simulink model "gm_sampleModel1811_5_sub"  (R2023a)
settings: Solver=VariableStepAuto  StartTime=0.0  StopTime=10.0  RelTol=1e-3
libraries: simulink x5
settings Model: Creator=user1  LastModifiedBy=user1
settings OptimizationCC: BlockReduction=off  ConditionallyExecuteInputs=off
settings DebuggingCC: InheritedTsInSrcMsg=none

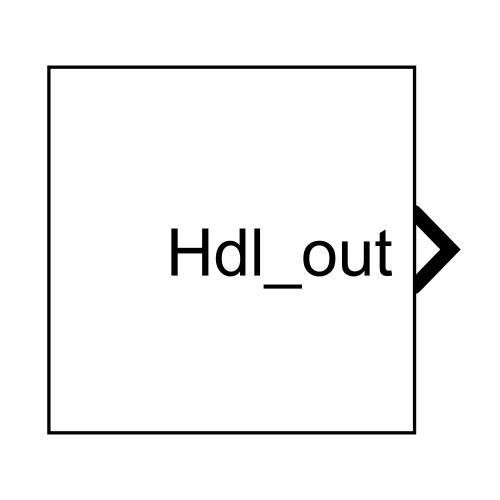
[thumbnail: Simulink's stored preview of the top-level diagram]
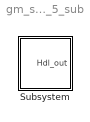
== system gm_sampleModel1811_5_sub ==
  Subsystem : Subsystem

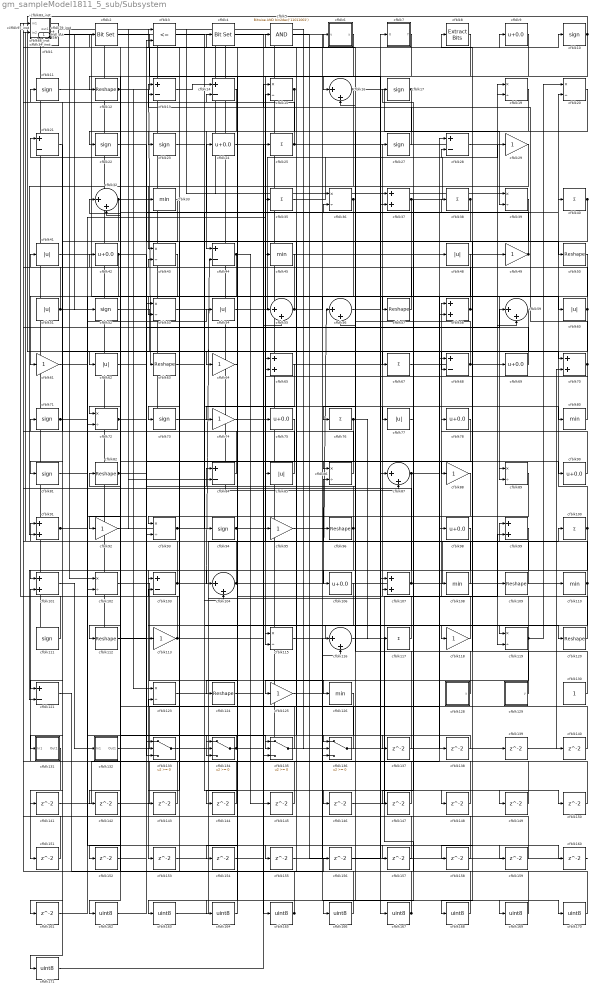
== system gm_sampleModel1811_5_sub/Subsystem ==
  cfblk1 : simulink/Logic and Bit Operations/Detect Decrease  vinit=0.0  OutDataTypeStr=uint8
      settings: LibrarySourceBlock=|
      | hdlsllib/Logic and Bit
      | Operations/Detect
      | Decrease
  cfblk{10..11,17,22..23,27,52,71,73,81,94,111} (12 alike) : Signum
  cfblk{25,35,38,40,67,76,100,117} (8 alike) : Sum  Inputs=+  OutDataTypeStr=uint8
  cfblk{37,58,65,70,91,99,101,107} (8 alike) : Sum  OutDataTypeStr=uint8
  cfblk{15,19..20,36,39,43,53,72,86,89,93,102,115,119,123} (15 alike) : Product  Inputs=*/  OutDataTypeStr=uint8  RndMeth=Zero  SaturateOnIntegerOverflow=on
  cfblk{13..14,21,28,44,68,84,103,121} (9 alike) : Sum  Inputs=+-  OutDataTypeStr=uint8
  cfblk{16,32,55..56,59,87,104,116} (8 alike) : Sum  Inputs=|++  OutDataTypeStr=uint8
  cfblk105_inst : Subsystem
  cfblk{9,24,42,69,75,78,90,98,106} (9 alike) : Bias  Bias=0.0  SaturateOnIntegerOverflow=off
  cfblk{33,45,80,108,110,126} (6 alike) : MinMax  OutDataTypeStr=uint8
  cfblk{12,50,57,63,82,96,109,112,120,124} (10 alike) : Reshape
  cfblk{29,49,61,64,74,88,92,95,113,118,125} (11 alike) : Gain  OutDataTypeStr=uint8
  cfblk114_inst : Subsystem
  cfblk122_inst : Subsystem
  cfblk128 : Subsystem  mask(Counter Free-Running){NumBits=double(16), tsamp=double(-1)}
      mask prompts: NumBits "Simulink:masks:NumberOfBits_MP"; tsamp "Simulink:masks:SampleTime_MP"
      mask help: Simulink:masks:CounterFreeRunning_MD
  cfblk129 : Subsystem  mask(Counter Limited){uplimit=double(7), tsamp=double(-1)}
      mask prompts: uplimit "Simulink:masks:UpperLimit_MP"; tsamp "Simulink:masks:SampleTime_MP"
      mask help: Simulink:masks:CounterLimited_MD
      mask init:
      | nbits = double(8);
      | tsamp = double(-1);
      | uplimit = double(7);
  cfblk130 : Constant  OutDataTypeStr=uint8  SampleTime=-1
  cfblk131 : Subsystem
  cfblk132 : Subsystem
  cfblk{133..136} (4 alike) : Switch  OutDataTypeStr=uint8  SaturateOnIntegerOverflow=off  InputSameDT=off
  cfblk{137..161} (25 alike) : Delay  SampleTime=1
  cfblk{162..171} (10 alike) : DataTypeConversion  OutDataTypeStr=uint8  SaturateOnIntegerOverflow=off  RndMeth=Floor
  cfblk18_inst : Subsystem
  cfblk2 : simulink/Logic and Bit Operations/Bit Set  iBit=0
      settings: LibrarySourceBlock=|
      | hdlsllib/Logic and Bit
      | Operations/Bit Set
  cfblk26_inst : Subsystem
  cfblk3 : RelationalOperator  Operator=<=  OutDataTypeStr=boolean  InputSameDT=off
  cfblk30_inst : Subsystem
  cfblk31_inst : Subsystem
  cfblk34_inst : Subsystem
  cfblk4 : simulink/Logic and Bit Operations/Bit Set  iBit=0
      settings: LibrarySourceBlock=|
      | hdlsllib/Logic and Bit
      | Operations/Bit Set
  cfblk{41,48,51,54,60,62,77,85} (8 alike) : Abs  OutDataTypeStr=uint8  SaturateOnIntegerOverflow=off
  cfblk5 : simulink/Logic and Bit Operations/Bitwise Operator  logicop=AND  UseBitMask=on  BitMask=bin2dec('11011001')  BitMaskRealWorld=Stored Integer
      settings: LibrarySourceBlock=|
      | hdlsllib/Logic and Bit
      | Operations/Bitwise
      | Operator
  cfblk6 : Subsystem  mask(Compare To Zero){relop=<=, OutDataTypeStr=uint8, ZeroCross=on}
      mask prompts: relop "Simulink:masks:Operator_MP"; OutDataTypeStr "Simulink:masks:OutputDataType_MP"; ZeroCross "Simulink:masks:EnableZerocrossingDetection_MP"
      mask help: Simulink:masks:CompareToZero_MD
      mask init:
      | OutDataTypeStr = 'uint8';
      | ZeroCross = 'on';
      | blkName = 'sampleModel1811_5_sub/Subsystem/cfblk6';
      | relop = '<=';
      | setValue = 'fixdt(0, 8)';
      mask TypeOptions relop: == | ~= | < | <= | >= | >
      mask TypeOptions OutDataTypeStr: Simulink:masks:uint8 | Simulink:masks:boolean
      mask Callback ZeroCross: sl('zeroCrossEnable', gcbh);
      mask Display: disp([relop,' 0'])
  cfblk66_inst : Subsystem
  cfblk7 : Subsystem  mask(Detect Fall Nonpositive){vinit=double(0), InputProcessing=Elements as channels (sample based), OutDataTypeStr=uint8}
      mask prompts: vinit "Simulink:masks:InitialCondition_MP"; InputProcessing "Simulink:masks:InputProcessing_MP"; OutDataTypeStr "Simulink:masks:OutputDataType_MP"
      mask help: Simulink:masks:DetectFallNonpositive_MD
      mask init:
      | InputProcessing = 'Elements as channels (sample based)';
      | OutDataTypeStr = 'uint8';
      | vinit = double(0);
      mask TypeOptions InputProcessing: Simulink:masks:ColumnsAsChannelsFrameBased | Simulink:masks:ElementsAsChannelsSampleBased
      mask TypeOptions OutDataTypeStr: Simulink:masks:uint8 | Simulink:masks:boolean
      mask Display: fprintf('U <= 0\n&  NOT\nU/z <= 0')
  cfblk79_inst : Subsystem
  cfblk8 : simulink/Logic and Bit Operations/Extract Bits  bitsToExtract=Upper half  numBits=8  bitIdxRange=[0 7]  outScalingMode=Preserve fixed-point scaling
      settings: LibrarySourceBlock=|
      | hdlsllib/Logic and Bit
      | Operations/Extract Bits
  cfblk83_inst : Subsystem
  cfblk97_inst : Subsystem
  Hdl_out : Outport  OutDataTypeStr=uint8  SampleTime=1
  wires:
  cfblk1/1 -> cfblk52/1, cfblk89/2
  cfblk10/1 -> cfblk62/1, cfblk115/2
  cfblk100/1 -> cfblk20/2, cfblk153/1
  cfblk101/1 -> cfblk132/1(In1)
  cfblk102/1 -> cfblk126/1
  cfblk103/1 -> cfblk44/2, cfblk31_inst/2(in2)
  cfblk104/1 -> cfblk56/1, cfblk18_inst/2(in2)
  cfblk105_inst/1(out1) -> cfblk122_inst/2(in2)
  cfblk106/1 -> cfblk113/1
  cfblk107/1 -> cfblk26_inst/2(in2), cfblk100/1
  cfblk108/1 -> cfblk15/2
  cfblk109/1 -> cfblk91/1
  cfblk11/1 -> cfblk109/1
  cfblk110/1 -> cfblk56/2, cfblk86/2, cfblk125/1
  cfblk111/1 -> cfblk83_inst/1(in1)
  cfblk112/1 -> cfblk10/1
  cfblk113/1 -> cfblk105_inst/2(in2), cfblk157/1, Hdl_out/1
  cfblk114_inst/1(out1) -> cfblk75/1, cfblk66_inst/2(in2), cfblk49/1
  cfblk115/1 -> cfblk118/1
  cfblk116/1 -> cfblk163/1
  cfblk117/1 -> cfblk27/1
  cfblk118/1 -> cfblk58/1
  cfblk119/1 -> cfblk135/2, cfblk107/2, cfblk20/1
  cfblk12/1 -> cfblk63/1, cfblk123/1, cfblk6/1(u)
  cfblk120/1 -> cfblk71/1
  cfblk121/1 -> cfblk156/1
  cfblk122_inst/1(out1) -> cfblk94/1, cfblk37/1
  cfblk123/1 -> cfblk99/1
  cfblk124/1 -> cfblk25/1
  cfblk125/1 -> cfblk116/2
  cfblk126/1 -> cfblk152/1
  cfblk128/1(y) -> cfblk84/1
  cfblk129/1(y) -> cfblk78/1
  cfblk13/1 -> cfblk14/1
  cfblk130/1 -> cfblk16/2
  cfblk131/1(Out1) -> cfblk151/1
  cfblk132/1(Out1) -> cfblk108/1
  cfblk133/1 -> cfblk85/1
  cfblk134/1 -> cfblk133/2, cfblk160/1
  cfblk135/1 -> cfblk43/2
  cfblk136/1 -> cfblk32/1
  cfblk137/1 -> cfblk97_inst/2(in2)
  cfblk138/1 -> cfblk136/1
  cfblk139/1 -> cfblk70/2
  cfblk14/1 -> cfblk72/1
  cfblk140/1 -> cfblk123/2
  cfblk141/1 -> cfblk28/1
  cfblk142/1 -> cfblk116/1
  cfblk143/1 -> cfblk83_inst/2(in2)
  cfblk144/1 -> cfblk32/2
  cfblk145/1 -> cfblk30_inst/2(in2)
  cfblk146/1 -> cfblk99/2
  cfblk147/1 -> cfblk101/2
  cfblk148/1 -> cfblk34_inst/2(in2)
  cfblk149/1 -> cfblk122_inst/1(in1)
  cfblk15/1 -> cfblk22/1, cfblk64/1
  cfblk150/1 -> cfblk14/2
  cfblk151/1 -> cfblk26_inst/1(in1)
  cfblk152/1 -> cfblk59/1
  cfblk153/1 -> cfblk107/1
  cfblk154/1 -> cfblk55/2
  cfblk155/1 -> cfblk136/3
  cfblk156/1 -> cfblk87/1
  cfblk157/1 -> cfblk3/1
  cfblk158/1 -> cfblk13/1
  cfblk159/1 -> cfblk79_inst/2(in2)
  cfblk16/1 -> cfblk43/1, cfblk39/2
  cfblk160/1 -> cfblk1/1
  cfblk161/1 -> cfblk72/2
  cfblk162/1 -> cfblk9/1
  cfblk163/1 -> cfblk7/1(U)
  cfblk164/1 -> cfblk4/1
  cfblk165/1 -> cfblk34_inst/1(in1), cfblk114_inst/1(in1)
  cfblk166/1 -> cfblk2/1
  cfblk167/1 -> cfblk82/1, cfblk133/1, cfblk103/2
  cfblk168/1 -> cfblk5/1
  cfblk169/1 -> cfblk17/1
  cfblk17/1 -> cfblk37/2, cfblk76/1
  cfblk170/1 -> cfblk97_inst/1(in1)
  cfblk171/1 -> cfblk95/1
  cfblk18_inst/1(out1) -> cfblk39/1
  cfblk19/1 -> cfblk44/1
  cfblk2/1 -> cfblk167/1
  cfblk20/1 -> cfblk23/1
  cfblk21/1 -> cfblk81/1
  cfblk22/1 -> cfblk50/1
  cfblk23/1 -> cfblk104/2
  cfblk24/1 -> cfblk89/1
  cfblk25/1 -> cfblk90/1, cfblk79_inst/1(in1)
  cfblk26_inst/1(out1) -> cfblk84/2
  cfblk27/1 -> cfblk15/1
  cfblk28/1 -> cfblk119/2
  cfblk29/1 -> cfblk91/2
  cfblk3/1 -> cfblk65/1
  cfblk30_inst/1(out1) -> cfblk111/1, cfblk102/1
  cfblk31_inst/1(out1) -> cfblk105_inst/1(in1), cfblk29/1
  cfblk32/1 -> cfblk161/1, cfblk33/1
  cfblk33/1 -> cfblk171/1
  cfblk34_inst/1(out1) -> cfblk69/1
  cfblk35/1 -> cfblk28/2
  cfblk36/1 -> cfblk102/2, cfblk131/1(In1)
  cfblk37/1 -> cfblk57/1, cfblk19/2, cfblk147/1
  cfblk38/1 -> cfblk103/1, cfblk115/1
  cfblk39/1 -> cfblk68/2
  cfblk4/1 -> cfblk165/1
  cfblk40/1 -> cfblk96/1, cfblk106/1
  cfblk41/1 -> cfblk98/1
  cfblk42/1 -> cfblk60/1, cfblk59/2, cfblk134/3, cfblk121/1, cfblk61/1
  cfblk43/1 -> cfblk141/1
  cfblk44/1 -> cfblk73/1, cfblk145/1, cfblk144/1
  cfblk45/1 -> cfblk74/1
  cfblk48/1 -> cfblk136/2
  cfblk49/1 -> cfblk24/1, cfblk21/1
  cfblk5/1 -> cfblk169/1
  cfblk50/1 -> cfblk93/1
  cfblk51/1 -> cfblk114_inst/2(in2), cfblk67/1
  cfblk52/1 -> cfblk70/1
  cfblk53/1 -> cfblk138/1
  cfblk54/1 -> cfblk19/1
  cfblk55/1 -> cfblk58/2, cfblk53/2
  cfblk56/1 -> cfblk80/1
  cfblk57/1 -> cfblk45/1
  cfblk58/1 -> cfblk42/1, cfblk168/1
  cfblk59/1 -> cfblk101/1
  cfblk6/1(y) -> cfblk104/1
  cfblk60/1 -> cfblk18_inst/1(in1), cfblk158/1
  cfblk61/1 -> cfblk159/1
  cfblk62/1 -> cfblk86/1
  cfblk63/1 -> cfblk77/1
  cfblk64/1 -> cfblk164/1
  cfblk65/1 -> cfblk124/1
  cfblk66_inst/1(out1) -> cfblk31_inst/1(in1), cfblk36/1
  cfblk67/1 -> cfblk120/1
  cfblk68/1 -> cfblk41/1, cfblk88/1
  cfblk69/1 -> cfblk30_inst/1(in1)
  cfblk7/1(Y) -> cfblk162/1
  cfblk70/1 -> cfblk65/2, cfblk13/2
  cfblk71/1 -> cfblk93/2, cfblk35/1
  cfblk72/1 -> cfblk3/2, cfblk38/1
  cfblk73/1 -> cfblk146/1
  cfblk74/1 -> cfblk148/1
  cfblk75/1 -> cfblk92/1
  cfblk76/1 -> cfblk134/1, cfblk117/1
  cfblk77/1 -> cfblk137/1
  cfblk78/1 -> cfblk135/3
  cfblk79_inst/1(out1) -> cfblk87/2
  cfblk8/1 -> cfblk16/1
  cfblk80/1 -> cfblk68/1
  cfblk81/1 -> cfblk155/1
  cfblk82/1 -> cfblk133/3, cfblk112/1
  cfblk83_inst/1(out1) -> cfblk51/1, cfblk21/2, cfblk140/1, cfblk139/1
  cfblk84/1 -> cfblk66_inst/1(in1)
  cfblk85/1 -> cfblk11/1
  cfblk86/1 -> cfblk55/1
  cfblk87/1 -> cfblk48/1, cfblk134/2
  cfblk88/1 -> cfblk143/1
  cfblk89/1 -> cfblk154/1
  cfblk9/1 -> cfblk12/1
  cfblk90/1 -> cfblk8/1
  cfblk91/1 -> cfblk54/1, cfblk135/1
  cfblk92/1 -> cfblk40/1
  cfblk93/1 -> cfblk36/2, cfblk119/1
  cfblk94/1 -> cfblk150/1, cfblk149/1
  cfblk95/1 -> cfblk170/1
  cfblk96/1 -> cfblk121/2, cfblk53/1
  cfblk97_inst/1(out1) -> cfblk110/1
  cfblk98/1 -> cfblk142/1
  cfblk99/1 -> cfblk166/1

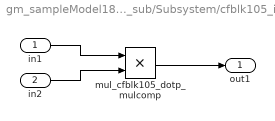
== system gm_sampleModel1811_5_sub/Subsystem/cfblk105_inst ==
  in1 : Inport  OutDataTypeStr=uint8  SampleTime=1
  in2 : Inport  Port=2  OutDataTypeStr=uint8  SampleTime=1
  mul_cfblk105_dotp_mulcomp : Product  Inputs=**  OutDataTypeStr=uint8  SampleTime=1
  out1 : Outport  OutDataTypeStr=uint8  SampleTime=1
  wires:
  in1/1 -> mul_cfblk105_dotp_mulcomp/1
  in2/1 -> mul_cfblk105_dotp_mulcomp/2
  mul_cfblk105_dotp_mulcomp/1 -> out1/1

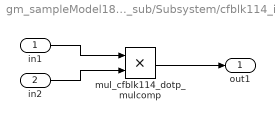
== system gm_sampleModel1811_5_sub/Subsystem/cfblk114_inst ==
  in1 : Inport  OutDataTypeStr=uint8  SampleTime=1
  in2 : Inport  Port=2  OutDataTypeStr=uint8  SampleTime=1
  mul_cfblk114_dotp_mulcomp : Product  Inputs=**  OutDataTypeStr=uint8  SampleTime=1
  out1 : Outport  OutDataTypeStr=uint8  SampleTime=1
  wires:
  in1/1 -> mul_cfblk114_dotp_mulcomp/1
  in2/1 -> mul_cfblk114_dotp_mulcomp/2
  mul_cfblk114_dotp_mulcomp/1 -> out1/1

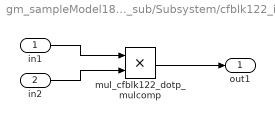
== system gm_sampleModel1811_5_sub/Subsystem/cfblk122_inst ==
  in1 : Inport  OutDataTypeStr=uint8  SampleTime=1
  in2 : Inport  Port=2  OutDataTypeStr=uint8  SampleTime=1
  mul_cfblk122_dotp_mulcomp : Product  Inputs=**  OutDataTypeStr=uint8  SampleTime=1
  out1 : Outport  OutDataTypeStr=uint8  SampleTime=1
  wires:
  in1/1 -> mul_cfblk122_dotp_mulcomp/1
  in2/1 -> mul_cfblk122_dotp_mulcomp/2
  mul_cfblk122_dotp_mulcomp/1 -> out1/1

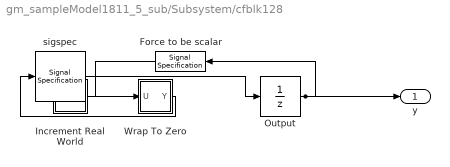
== system gm_sampleModel1811_5_sub/Subsystem/cfblk128 ==
  Force to be scalar : SignalSpecification  DisableCoverage=on  Dimensions=1
  Increment Real World : Subsystem  mask(Real World Value Increment){}
      mask help: Simulink:masks:RealWorldValueIncrement_MD
      mask Display: disp('V++')
  Output : UnitDelay  InitialCondition=0.0  SampleTime=tsamp  HasFrameUpgradeWarning=on
  Wrap To Zero : Subsystem  mask(Wrap To Zero){Threshold=double(65535)}
      mask prompts: Threshold "Simulink:masks:Threshold_MP"
      mask help: Simulink:masks:WrapToZero_MD
  sigspec : SignalSpecification  OutDataTypeStr=uint16  Dimensions=1
  y : Outport  SampleTime=1
  wires:
  Force to be scalar/1 -> Increment Real World/1(u)
  Increment Real World/1(y) -> Wrap To Zero/1(U)
  Output/1 -> Force to be scalar/1, y/1
  Wrap To Zero/1(Y) -> sigspec/1
  sigspec/1 -> Output/1

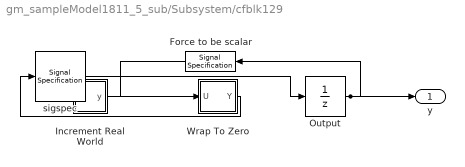
== system gm_sampleModel1811_5_sub/Subsystem/cfblk129 ==
  Force to be scalar : SignalSpecification  DisableCoverage=on  Dimensions=1
  Increment Real World : Subsystem  mask(Real World Value Increment){}
      mask help: Simulink:masks:RealWorldValueIncrement_MD
      mask Display: disp('V++')
  Output : UnitDelay  InitialCondition=0.0  SampleTime=tsamp  HasFrameUpgradeWarning=on
  Wrap To Zero : Subsystem  mask(Wrap To Zero){Threshold=double(7)}
      mask prompts: Threshold "Simulink:masks:Threshold_MP"
      mask help: Simulink:masks:WrapToZero_MD
  sigspec : SignalSpecification  OutDataTypeStr=uint8  Dimensions=1
  y : Outport  SampleTime=1
  wires:
  Force to be scalar/1 -> Increment Real World/1(u)
  Increment Real World/1(y) -> Wrap To Zero/1(U)
  Output/1 -> Force to be scalar/1, y/1
  Wrap To Zero/1(Y) -> sigspec/1
  sigspec/1 -> Output/1

== system gm_sampleModel1811_5_sub/Subsystem/cfblk131 ==
  In1 : Inport  OutDataTypeStr=uint8  PortDimensions=1  SampleTime=1
  Out1 : Outport  SampleTime=1
  wires:
  In1/1 -> Out1/1

== system gm_sampleModel1811_5_sub/Subsystem/cfblk132 ==
  In1 : Inport  OutDataTypeStr=uint8  PortDimensions=1  SampleTime=1
  Out1 : Outport  SampleTime=1
  wires:
  In1/1 -> Out1/1

== system gm_sampleModel1811_5_sub/Subsystem/cfblk18_inst ==
  in1 : Inport  OutDataTypeStr=uint8  SampleTime=1
  in2 : Inport  Port=2  OutDataTypeStr=uint8  SampleTime=1
  mul_cfblk18_dotp_mulcomp : Product  Inputs=**  OutDataTypeStr=uint8  SampleTime=1
  out1 : Outport  OutDataTypeStr=uint8  SampleTime=1
  wires:
  in1/1 -> mul_cfblk18_dotp_mulcomp/1
  in2/1 -> mul_cfblk18_dotp_mulcomp/2
  mul_cfblk18_dotp_mulcomp/1 -> out1/1

== system gm_sampleModel1811_5_sub/Subsystem/cfblk26_inst ==
  in1 : Inport  OutDataTypeStr=uint8  SampleTime=1
  in2 : Inport  Port=2  OutDataTypeStr=uint8  SampleTime=1
  mul_cfblk26_dotp_mulcomp : Product  Inputs=**  OutDataTypeStr=uint8  SampleTime=1
  out1 : Outport  OutDataTypeStr=uint8  SampleTime=1
  wires:
  in1/1 -> mul_cfblk26_dotp_mulcomp/1
  in2/1 -> mul_cfblk26_dotp_mulcomp/2
  mul_cfblk26_dotp_mulcomp/1 -> out1/1

== system gm_sampleModel1811_5_sub/Subsystem/cfblk30_inst ==
  in1 : Inport  OutDataTypeStr=uint8  SampleTime=1
  in2 : Inport  Port=2  OutDataTypeStr=uint8  SampleTime=1
  mul_cfblk30_dotp_mulcomp : Product  Inputs=**  OutDataTypeStr=uint8  SampleTime=1
  out1 : Outport  OutDataTypeStr=uint8  SampleTime=1
  wires:
  in1/1 -> mul_cfblk30_dotp_mulcomp/1
  in2/1 -> mul_cfblk30_dotp_mulcomp/2
  mul_cfblk30_dotp_mulcomp/1 -> out1/1

== system gm_sampleModel1811_5_sub/Subsystem/cfblk31_inst ==
  in1 : Inport  OutDataTypeStr=uint8  SampleTime=1
  in2 : Inport  Port=2  OutDataTypeStr=uint8  SampleTime=1
  mul_cfblk31_dotp_mulcomp : Product  Inputs=**  OutDataTypeStr=uint8  SampleTime=1
  out1 : Outport  OutDataTypeStr=uint8  SampleTime=1
  wires:
  in1/1 -> mul_cfblk31_dotp_mulcomp/1
  in2/1 -> mul_cfblk31_dotp_mulcomp/2
  mul_cfblk31_dotp_mulcomp/1 -> out1/1

== system gm_sampleModel1811_5_sub/Subsystem/cfblk34_inst ==
  in1 : Inport  OutDataTypeStr=uint8  SampleTime=1
  in2 : Inport  Port=2  OutDataTypeStr=uint8  SampleTime=1
  mul_cfblk34_dotp_mulcomp : Product  Inputs=**  OutDataTypeStr=uint8  SampleTime=1
  out1 : Outport  OutDataTypeStr=uint8  SampleTime=1
  wires:
  in1/1 -> mul_cfblk34_dotp_mulcomp/1
  in2/1 -> mul_cfblk34_dotp_mulcomp/2
  mul_cfblk34_dotp_mulcomp/1 -> out1/1

== system gm_sampleModel1811_5_sub/Subsystem/cfblk6 ==
  u : Inport  OutDataTypeStr=uint8  SampleTime=1
  Compare : RelationalOperator  Operator=<=  OutDataTypeStr=fixdt(0, 8)
  Constant : Constant  DisableCoverage=on  Value=0  OutDataTypeStr=Inherit: Inherit via back propagation  SampleTime=-1  PreserveConstantTs=on
  y : Outport  SampleTime=1
  wires:
  u/1 -> Compare/1
  Compare/1 -> y/1
  Constant/1 -> Compare/2

== system gm_sampleModel1811_5_sub/Subsystem/cfblk66_inst ==
  in1 : Inport  OutDataTypeStr=uint8  SampleTime=1
  in2 : Inport  Port=2  OutDataTypeStr=uint8  SampleTime=1
  mul_cfblk66_dotp_mulcomp : Product  Inputs=**  OutDataTypeStr=uint8  SampleTime=1
  out1 : Outport  OutDataTypeStr=uint8  SampleTime=1
  wires:
  in1/1 -> mul_cfblk66_dotp_mulcomp/1
  in2/1 -> mul_cfblk66_dotp_mulcomp/2
  mul_cfblk66_dotp_mulcomp/1 -> out1/1

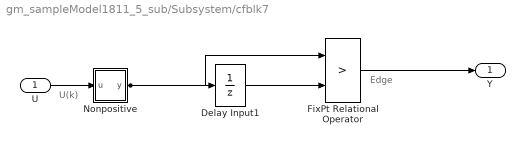
== system gm_sampleModel1811_5_sub/Subsystem/cfblk7 ==
  note: U(k)
  note: Edge
  U : Inport  OutDataTypeStr=uint8  SampleTime=1
  Delay Input1 : UnitDelay  Description=Store in Global RAM  DisableCoverage=on  InitialCondition=vinit  SampleTime=-1  HasFrameUpgradeWarning=on
  FixPt Relational Operator : RelationalOperator  Operator=>  OutDataTypeStr=fixdt(0, 8)  ZeroCross=off  InputSameDT=off
  Nonpositive : Subsystem  mask(Compare To Zero){relop=<=, OutDataTypeStr=boolean, ZeroCross=off}
      mask prompts: relop "Simulink:masks:Operator_MP"; OutDataTypeStr "Simulink:masks:OutputDataType_MP"; ZeroCross "Simulink:masks:EnableZerocrossingDetection_MP"
      mask help: Simulink:masks:CompareToZero_MD
      mask init:
      | OutDataTypeStr = 'boolean';
      | ZeroCross = 'off';
      | blkName = 'sampleModel1811_5_sub/Subsystem/cfblk7/Nonpositive';
      | relop = '<=';
      | setValue = 'boolean';
      mask TypeOptions relop: == | ~= | < | <= | >= | >
      mask TypeOptions OutDataTypeStr: Simulink:masks:uint8 | Simulink:masks:boolean
      mask Callback ZeroCross: sl('zeroCrossEnable', gcbh);
      mask Display: disp([relop,' 0'])
  Y : Outport  SampleTime=1
  wires:
  U/1 -> Nonpositive/1(u)
  Delay Input1/1 -> FixPt Relational Operator/2
  FixPt Relational Operator/1 -> Y/1
  Nonpositive/1(y) -> FixPt Relational Operator/1, Delay Input1/1

== system gm_sampleModel1811_5_sub/Subsystem/cfblk79_inst ==
  in1 : Inport  OutDataTypeStr=uint8  SampleTime=1
  in2 : Inport  Port=2  OutDataTypeStr=uint8  SampleTime=1
  mul_cfblk79_dotp_mulcomp : Product  Inputs=**  OutDataTypeStr=uint8  SampleTime=1
  out1 : Outport  OutDataTypeStr=uint8  SampleTime=1
  wires:
  in1/1 -> mul_cfblk79_dotp_mulcomp/1
  in2/1 -> mul_cfblk79_dotp_mulcomp/2
  mul_cfblk79_dotp_mulcomp/1 -> out1/1

== system gm_sampleModel1811_5_sub/Subsystem/cfblk83_inst ==
  in1 : Inport  OutDataTypeStr=uint8  SampleTime=1
  in2 : Inport  Port=2  OutDataTypeStr=uint8  SampleTime=1
  mul_cfblk83_dotp_mulcomp : Product  Inputs=**  OutDataTypeStr=uint8  SampleTime=1
  out1 : Outport  OutDataTypeStr=uint8  SampleTime=1
  wires:
  in1/1 -> mul_cfblk83_dotp_mulcomp/1
  in2/1 -> mul_cfblk83_dotp_mulcomp/2
  mul_cfblk83_dotp_mulcomp/1 -> out1/1

== system gm_sampleModel1811_5_sub/Subsystem/cfblk97_inst ==
  in1 : Inport  OutDataTypeStr=uint8  SampleTime=1
  in2 : Inport  Port=2  OutDataTypeStr=uint8  SampleTime=1
  mul_cfblk97_dotp_mulcomp : Product  Inputs=**  OutDataTypeStr=uint8  SampleTime=1
  out1 : Outport  OutDataTypeStr=uint8  SampleTime=1
  wires:
  in1/1 -> mul_cfblk97_dotp_mulcomp/1
  in2/1 -> mul_cfblk97_dotp_mulcomp/2
  mul_cfblk97_dotp_mulcomp/1 -> out1/1

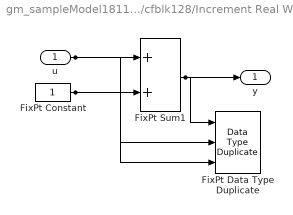
== system gm_sampleModel1811_5_sub/Subsystem/cfblk128/Increment Real World ==
  u : Inport  OutDataTypeStr=uint16  SampleTime=1
  FixPt Constant : Constant  DisableCoverage=on  OutDataTypeStr=Inherit: Inherit via back propagation  SampleTime=-1
  FixPt Data Type Duplicate : DataTypeDuplicate  DisableCoverage=on  NumInputPorts=3
  FixPt Sum1 : Sum  InputSameDT=on  OutDataTypeStr=Inherit: Inherit via back propagation  LockScale=on
  y : Outport  SampleTime=1
  wires:
  u/1 -> FixPt Sum1/1, FixPt Data Type Duplicate/2
  FixPt Constant/1 -> FixPt Sum1/2, FixPt Data Type Duplicate/3
  FixPt Sum1/1 -> FixPt Data Type Duplicate/1, y/1

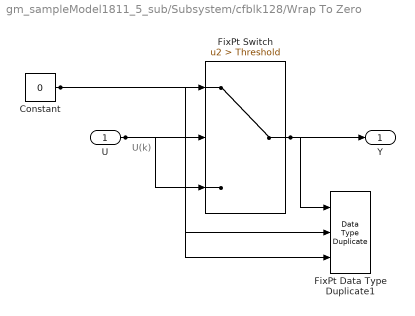
== system gm_sampleModel1811_5_sub/Subsystem/cfblk128/Wrap To Zero ==
  note: U(k)
  U : Inport  OutDataTypeStr=uint16  SampleTime=1
  Constant : Constant  DisableCoverage=on  Value=0  OutDataTypeStr=Inherit: Inherit via back propagation  SampleTime=-1
  FixPt Data Type Duplicate1 : DataTypeDuplicate  DisableCoverage=on  NumInputPorts=3
  FixPt Switch : Switch  Criteria=u2 > Threshold  Threshold=Threshold  OutDataTypeStr=Inherit: Inherit via back propagation  ZeroCross=off  SaturateOnIntegerOverflow=off  InputSameDT=off
  Y : Outport  SampleTime=1
  wires:
  U/1 -> FixPt Switch/3, FixPt Switch/2, FixPt Data Type Duplicate1/2
  Constant/1 -> FixPt Switch/1, FixPt Data Type Duplicate1/3
  FixPt Switch/1 -> FixPt Data Type Duplicate1/1, Y/1

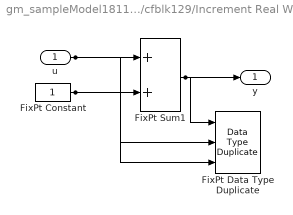
== system gm_sampleModel1811_5_sub/Subsystem/cfblk129/Increment Real World ==
  u : Inport  OutDataTypeStr=uint8  SampleTime=1
  FixPt Constant : Constant  DisableCoverage=on  OutDataTypeStr=Inherit: Inherit via back propagation  SampleTime=-1
  FixPt Data Type Duplicate : DataTypeDuplicate  DisableCoverage=on  NumInputPorts=3
  FixPt Sum1 : Sum  InputSameDT=on  OutDataTypeStr=Inherit: Inherit via back propagation  LockScale=on
  y : Outport  SampleTime=1
  wires:
  u/1 -> FixPt Sum1/1, FixPt Data Type Duplicate/2
  FixPt Constant/1 -> FixPt Sum1/2, FixPt Data Type Duplicate/3
  FixPt Sum1/1 -> FixPt Data Type Duplicate/1, y/1

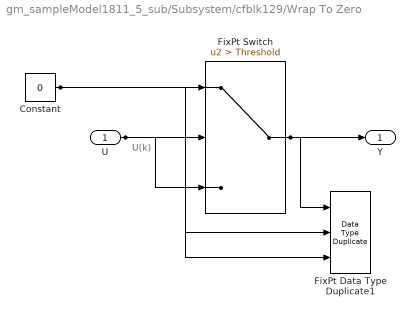
== system gm_sampleModel1811_5_sub/Subsystem/cfblk129/Wrap To Zero ==
  note: U(k)
  U : Inport  OutDataTypeStr=uint8  SampleTime=1
  Constant : Constant  DisableCoverage=on  Value=0  OutDataTypeStr=Inherit: Inherit via back propagation  SampleTime=-1
  FixPt Data Type Duplicate1 : DataTypeDuplicate  DisableCoverage=on  NumInputPorts=3
  FixPt Switch : Switch  Criteria=u2 > Threshold  Threshold=Threshold  OutDataTypeStr=Inherit: Inherit via back propagation  ZeroCross=off  SaturateOnIntegerOverflow=off  InputSameDT=off
  Y : Outport  SampleTime=1
  wires:
  U/1 -> FixPt Switch/3, FixPt Switch/2, FixPt Data Type Duplicate1/2
  Constant/1 -> FixPt Switch/1, FixPt Data Type Duplicate1/3
  FixPt Switch/1 -> FixPt Data Type Duplicate1/1, Y/1

== system gm_sampleModel1811_5_sub/Subsystem/cfblk7/Nonpositive ==
  u : Inport  OutDataTypeStr=uint8  SampleTime=1
  Compare : RelationalOperator  Operator=<=  OutDataTypeStr=boolean  ZeroCross=off
  Constant : Constant  DisableCoverage=on  Value=0  OutDataTypeStr=Inherit: Inherit via back propagation  SampleTime=-1  PreserveConstantTs=on
  y : Outport  SampleTime=1
  wires:
  u/1 -> Compare/1
  Compare/1 -> y/1
  Constant/1 -> Compare/2
